simulink model "environmentLib"  (R2020b)
settings: Solver=ode3  StartTime=0.0  StopTime=10.0  FixedStep=Ts  RelTol=1e-3  EnableMultiTasking=on
undefined symbols (not defined in the file): States, WMM2020
libraries: aerolibatmos2 x1, aerolibgravity2 x1
settings Model: Creator=dbell44  LastModifiedBy=dbell44
settings DebuggingCC: BusObjectLabelMismatch=none

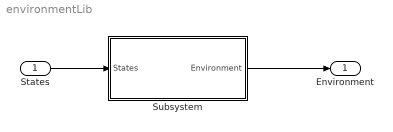
== system environmentLib ==
  States : Inport  OutDataTypeStr=Bus: StatesBus
  Subsystem : Subsystem
  Environment : Outport  OutDataTypeStr=Bus: EnvironmentBus
  wires:
  States/1 -> Subsystem/1(States)
  Subsystem/1(Environment) -> Environment/1

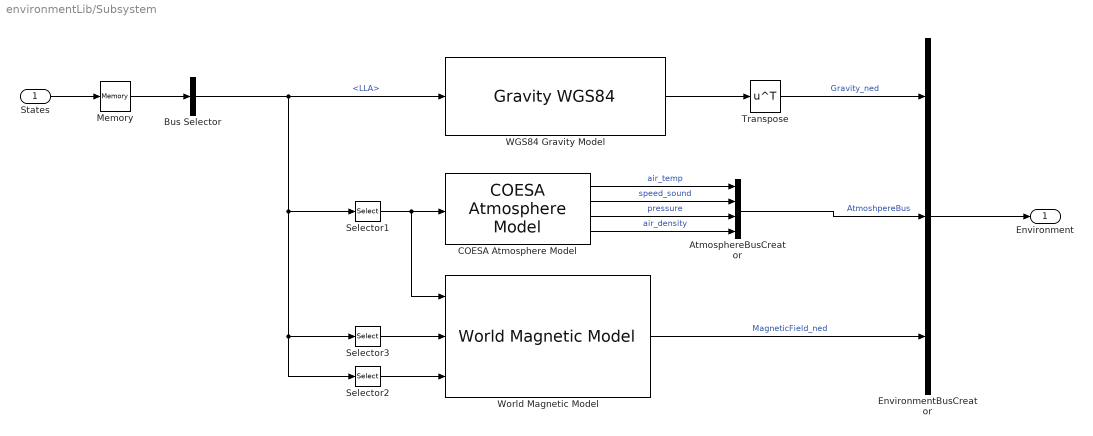
== system environmentLib/Subsystem ==
  States : Inport  OutDataTypeStr=Bus: StatesBus  Interpolate=off
  AtmosphereBusCreator : BusCreator  Inputs=4  OutDataTypeStr=Bus: AtmosphereBus
  Bus Selector : BusSelector  OutputSignals=LLA
  COESA Atmosphere Model : aerolibatmos2/COESA Atmosphere Model  units=Metric (MKS)  spec=1976 COESA-extended U.S. Standard Atmosphere  model=Profile  profile_var=High temperature  profile_percent=1%  profile_alt=5 km (16404 ft)  envelope_var=High temperature  envelope_percent=1%  action=Warning
  EnvironmentBusCreator : BusCreator  Inputs=3  OutDataTypeStr=Bus: EnvironmentBus
  Memory : Memory  InitialCondition=States  InheritSampleTime=on
  Selector1 : Selector  InputPortWidth=3  IndexOptions=Index vector (dialog)  Indices=[3]  OutputSizes=1
  Selector2 : Selector  InputPortWidth=3  IndexOptions=Index vector (dialog)  Indices=[2]  OutputSizes=1
  Selector3 : Selector  InputPortWidth=3  IndexOptions=Index vector (dialog)  Indices=[1]  OutputSizes=1
  Transpose : Math  Operator=transpose  SaturateOnIntegerOverflow=on
  "WGS84 Gravity Model  " : GravityWGS84
  World Magnetic Model : aerolibgravity2/World Magnetic Model  model=WMM2020 (2020-2025)  customFile='WMM2020.COF'  units=Metric (MKS)  time_in=off  month=January  day=1  year=2020  action=Error  h_out=off  dec_out=off  inc_out=off  ti_out=off
      settings: SourceProductBaseCode=AE
  Environment : Outport  OutDataTypeStr=Bus: EnvironmentBus
  wires:
  COESA Atmosphere Model/1 -> AtmosphereBusCreator/1  "air_temp"
  COESA Atmosphere Model/3 -> AtmosphereBusCreator/3  "pressure"
  Selector1/1 -> COESA Atmosphere Model/1, World Magnetic Model/1
  Selector3/1 -> World Magnetic Model/2
  "WGS84 Gravity Model  "/1 -> Transpose/1
  COESA Atmosphere Model/4 -> AtmosphereBusCreator/4  "air_density"
  AtmosphereBusCreator/1 -> EnvironmentBusCreator/2  "AtmoshpereBus"
  COESA Atmosphere Model/2 -> AtmosphereBusCreator/2  "speed_sound"
  Memory/1 -> Bus Selector/1
  Selector2/1 -> World Magnetic Model/3
  Transpose/1 -> EnvironmentBusCreator/1  "Gravity_ned"
  EnvironmentBusCreator/1 -> Environment/1
  World Magnetic Model/1 -> EnvironmentBusCreator/3  "MagneticField_ned"
  Bus Selector/1 -> Selector2/1, Selector3/1, Selector1/1, "WGS84 Gravity Model  "/1  "<LLA>"
  States/1 -> Memory/1
